simulink model "TCM64QAM_32QAM"  (Simulink 10.2)
settings: Solver=VariableStepDiscrete  StartTime=0.0  StopTime=1000  RelTol=1e-3  EnableMultiTasking=on
model workspace (MAT data in the model file):
  A = 1
  BER_exit = 0.0017398260174
  BER_th = 0.001
  K = 32
  M = 64
  N = 50
  P_TCM = 42
  P_UNCODED = 20.6666666667
  T = 1
  ber_TCM = [0.391236338113 0.382773488419 0.372666198737 0.362839667101 0.34830041111 0.338594204352 0.32505765567 0.309034392861 0.296741201243 0.281058858919 0.266339115612 0.248551087937 0.23457334804 0.215401584278 0.194144189311 0.138453825328 0.0571743708012 0.00563521508072 0.000521407801063 4.01082923895e-05]
  ber_UNCODED = [0.335246475352 0.314468553145 0.294510548945 0.272232776722 0.248595140486 0.22599740026 0.204779522048 0.183241675832 0.16104389561 0.140525947405 0.119748025197 0.10102989701 0.0794720527947 0.0601739826017 0.0424757524248 0.0288171182882 0.0175182481752 0.00995900409959 0.0048195180482 0.0017398260174]
  ber_tcm_bit_coded = [0.48089842575 0.489371302517 0.488168053745 0.487265617166 0.483605735486 0.484508172065 0.484056953775 0.483455329389 0.474029880678 0.474430963602 0.468715531936 0.456582773488 0.44745813697 0.426702095658 0.405444700692 0.320164443999 0.142986062368 0.0183495437682 0.000802165847789 0]
  ber_tcm_bit_uncoded = [0.350234149856 0.340341535072 0.326371459304 0.305454545455 0.28245363766 0.265181458857 0.235078627591 0.191129032258 0.17 0.133428860418 0.104998403066 0.0721370604148 0.0580141843972 0.0456842923795 0.0325443786982 0.0185420832576 0.00556319539942 0.00110539845758 0.000276048986147 5.01353654868e-05]
  coded_bit = 5
  coded_bit_conv = [5 6]
  codegen = [1  0  0  0  0  0; 0  1  0  0  0  0; 0  0  1  0  0  0; 0  0  0  1  0  0; 0  0  0  0  133  171]
  codegen_2 = [133 171]
  constlen = [1 1 1 1 7]
  constlen_2 = 7
  generator_c1 = 133
  generator_c2 = 171
  h = 22
  hh = 0
  hws = Simulink.ModelWorkspace
  i = 21
  k = 5
  label_coded = 'TCM64QAM'
  label_uncoded = '32QAM'
  list : struct (value not decoded)
  m = 6
  mapping_tcm = [-5-5i 3+3i -5+3i 3-5i -1-1i 7+7i -1+7i 7-1i -5-1i 3+7i -5+7i 3-1i -1-5i 7+3i -1+3i 7-5i -7-7i 1+1i -7+1i 1-7i -3-3i 5+5i -3+5i 5-3i -7-3i 1+5i -7+5i 1-3i -3-7i 5+1i -3+1i 5-7i -7-1i 1+7i -7+7i 1-1i -3-5i 5+3i -3+3i 5-5i -7-5i 1+3i -7+3i 1-5i -3-1i 5+7i -3+7i 5-1i -5-3i 3+5i -5+5i 3-3i -1-7i 7+1i -1+1i 7-7i -5-7i 3+1i -5+1i 3-7i -1-3i 7+5i -1+5i 7-3i]
  mdl_name = 'TCM64QAM_32QAM'
  mm = 0
  n = 10000
  num_states = 64
  register_length = 7
  seed = 210846
  snr = 20
  snr_start = 0
  snr_step = 1
  snr_vec = [0 1 2 3 4 5 6 7 8 9 10 11 12 13 14 15 16 17 18 19 20]
  ss = 0.721
  startTime = [2021 6 12 8 25 36.464]
  stepTime = [2021 6 12 8 25 56.984]
  step_dur = 0.721
  tb = 28
  tout = [9001 9002 9003 9004 9005 9006 9007 9008 9009 9010 9011 9012 ... (1000 elements, 1000x1)]
  trellis.numInputSymbols = 32
  trellis.numOutputSymbols = 64
  trellis.numStates = 64
  trellis.nextStates = [0 0 1 1 2 2 3 3 4 4 5 5 ... (2048 elements, 64x32)]
  trellis.outputs = [0 3 2 1 0 3 2 1 3 0 1 2 ... (2048 elements, 64x32)]
  trellis_2.numInputSymbols = 2
  trellis_2.numOutputSymbols = 4
  trellis_2.numStates = 64
  trellis_2.nextStates = [0  32; 0  32; 1  33; 1  33; 2  34; 2  34; 3  35; 3  35; 4  36; 4  36; 5  37; 5  37; 6  38; 6  38; 7  39; 7  39; 8  40; 8  40; 9  41; 9  41; 10  42; 10  42; 11  43; 11  43; 12  44; 12  44; 13  45; 13  45; 14  46; 14  46; 15  47; 15  47; 16  48; 16  48; 17  49; 17  49; 18  50; 18  50; 19  51; 19  51; 20  52; 20  52; 21  53; 21  53; 22  54; 22  54; 23  55; 23  55; 24  56; 24  56; 25  57; 25  57; 26  58; 26  58; 27  59; 27  59; 28  60; 28  60; 29  61; 29  61; 30  62; 30  62; 31  63; 31  63]
  trellis_2.outputs = [0  3; 3  0; 2  1; 1  2; 0  3; 3  0; 2  1; 1  2; 3  0; 0  3; 1  2; 2  1; 3  0; 0  3; 1  2; 2  1; 3  0; 0  3; 1  2; 2  1; 3  0; 0  3; 1  2; 2  1; 0  3; 3  0; 2  1; 1  2; 0  3; 3  0; 2  1; 1  2; 1  2; 2  1; 3  0; 0  3; 1  2; 2  1; 3  0; 0  3; 2  1; 1  2; 0  3; 3  0; 2  1; 1  2; 0  3; 3  0; 2  1; 1  2; 0  3; 3  0; 2  1; 1  2; 0  3; 3  0; 1  2; 2  1; 3  0; 0  3; 1  2; 2  1; 3  0; 0  3]
  uncoded_bit = [1 2 3 4]
undefined symbols (not defined in the file): Mnum
libraries: commsink2 x4, commutil2 x4, dspindex x4, commdigbbndam3 x3, commchan3 x2, commcnvcod2 x2, commdigbbndtcm2 x1, commrandsrc2 x1
settings Model: Creator=Diego  LastModifiedBy=diego
settings DataIOCC: LimitDataPoints=on
settings OptimizationCC: ExpressionDepthLimit=2147483647
settings DebuggingCC: SolverPrmCheckMsg=warning  StateNameClashWarn=warning
settings GRTTargetCC: CombineOutputUpdateFcns=on  GRTInterface=off

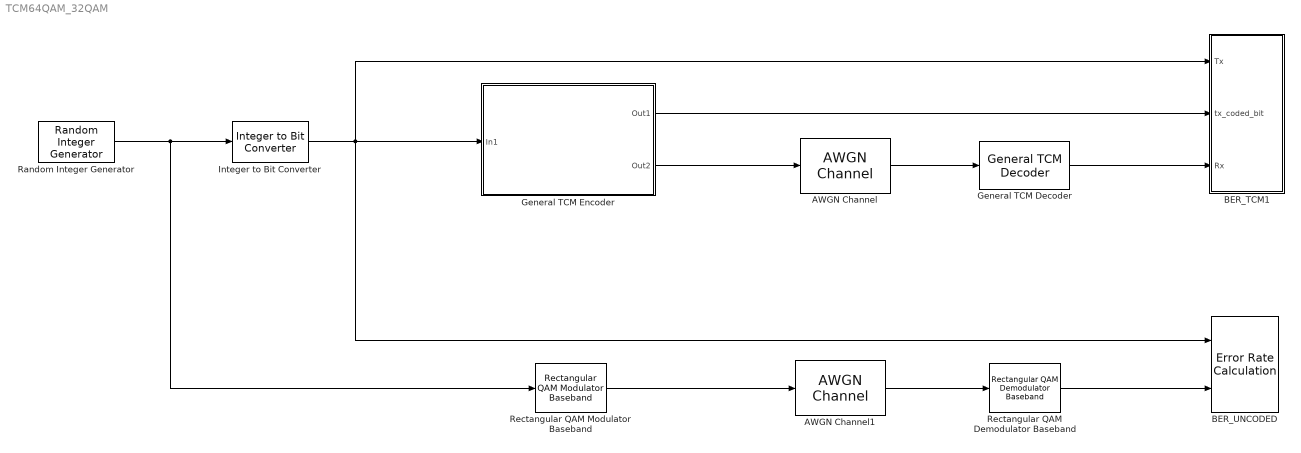
== system TCM64QAM_32QAM ==
  AWGN Channel : commchan3/AWGN Channel  InputProcessing=Columns as channels (frame based)  seed=seed  noiseMode="Signal to noise ratio  (Es/No)"  EbNodB=Eb_No  EsNodB=snr  SNRdB=snr  bitsPerSym=k  Ps=P_TCM  Tsym=T  variance=1
  AWGN Channel1 : commchan3/AWGN Channel  InputProcessing=Columns as channels (frame based)  seed=seed  noiseMode="Signal to noise ratio  (Es/No)"  EbNodB=Eb_No  EsNodB=snr  SNRdB=snr  bitsPerSym=k  Ps=P_UNCODED  Tsym=1  variance=1
  BER_TCM1 : Subsystem
  BER_UNCODED : commsink2/Error Rate Calculation  N=0  st_delay=0  cp_mode=Entire frame  subframe=[]  PMode=Workspace  WsName=ErrorVec_UNCODED  RsMode2=off  stop=off  numErr=100  maxBits=1e6
  General TCM Decoder : commdigbbndtcm2/General TCM Decoder  trellis=trellis  constpts=mapping_tcm  tbdepth=tb  opmode=Continuous  reset=off  outDtype=double
      settings: SourceProductBaseCode=CM
  General TCM Encoder : Subsystem  AncestorBlock=commdigbbndtcm2/General TCM Encoder  mask(General TCM Encoder){trellis=trellis, opMode=Continuous, constpts=mapping_tcm, outDtype=double}
      mask prompts: trellis "Trellis structure:"; opMode "Operation mode:"; constpts "Signal constellation:"; outDtype "Output data type"
      mask help:
      | Convolutionally encode binary data and perform signal mapping using the Signal constellation parameter, which expects complex constellation points in the set-partitioned order.
      |
      | The Trellis structure parameter must be a valid MATLAB trellis structure. To check if a structure is a valid trellis structure, use the istrellis function in MATLAB.
      mask init:
      | [constpts, Mnum, err, inPortLbl, rstPortLbl] = commblkgentcmenc(gcb, 'init', trellis, constpts);
      | if ~isempty(err.msg)
      | 	error(err.mmi,err.msg);
      | end
      mask Help: helpview(commbhelp)
      mask TypeOptions opMode: Continuous | Truncated (reset every frame) | Terminate trellis by appending bits | Reset on nonzero input via port
      mask TypeOptions outDtype: double | single
      mask Callback outDtype: commblkgentcmenc(gcb, 'cbDtype');
      mask Display:
      | disp('General\nTCM');
      | text(inPortLbl.x, inPortLbl.y, inPortLbl.str);
      | text(rstPortLbl.x, rstPortLbl.y, rstPortLbl.str);
  Integer to Bit Converter : commutil2/Integer to Bit Converter  nbits=k  signedInputValues=Unsigned  bitOrder=MSB first  outDtype=Inherit via internal rule
  Random Integer Generator : commrandsrc2/Random Integer Generator  mul=K  seed=seed  Ts=1  frameBased=off  sampPerFrame=frame  orient=off  outDataType=double
      settings: SourceProductBaseCode=CM
  Rectangular QAM Demodulator Baseband : commdigbbndam3/Rectangular QAM Demodulator Baseband  M=K  OutType=Bit  DecType=Hard decision  VarSource=Dialog  Variance=1  Dec=Gray  Mapping=[0:15]  PowType=Min. distance between symbols  MinDist=2  AvgPow=1  PeakPow=1  Ph=0  outDtype1=Inherit via internal rule  outDtype2=Inherit via internal rule  derotateFactorWordLen=16  derotateFactorDataTypeStr=Inherit: Same word length as input  derotateFactorLastDataTypeStr=Inherit: Same word length as input  denormFactorWordLen=16  denormFactorDataTypeStr=Inherit: Same word length as input  denormFactorLastDataTypeStr=Inherit: Same word length as input  prodOutWordLen=32  prodOutOverflowMode=Wrap  prodOutRoundingMode=Floor  prodOutOvFlMode=off  prodOutOvFlModeLastStrValue=off  sumWordLen=32
  Rectangular QAM Modulator Baseband : commdigbbndam3/Rectangular QAM Modulator Baseband  M=K  InType=Integer  Enc=Gray  Mapping=[0:15]  PowType=Min. distance between symbols  MinDist=2  AvgPow=1  PeakPow=1  Ph=0  outDtype=double  outWordLen=16  outUDDataType=sfix(16)  outFracLenMode=Best precision  outFracLen=15  outDataTypeStr=double  outLastDataTypeStr=double
  wires:
  Random Integer Generator/1 -> Integer to Bit Converter/1, Rectangular QAM Modulator Baseband/1
  Integer to Bit Converter/1 -> BER_UNCODED/1, General TCM Encoder/1(In1), BER_TCM1/1(Tx)
  General TCM Encoder/2(Out2) -> AWGN Channel/1
  AWGN Channel/1 -> General TCM Decoder/1
  Rectangular QAM Modulator Baseband/1 -> AWGN Channel1/1
  AWGN Channel1/1 -> Rectangular QAM Demodulator Baseband/1
  Rectangular QAM Demodulator Baseband/1 -> BER_UNCODED/2
  General TCM Decoder/1 -> BER_TCM1/3(Rx)
  General TCM Encoder/1(Out1) -> BER_TCM1/2(tx_coded_bit)

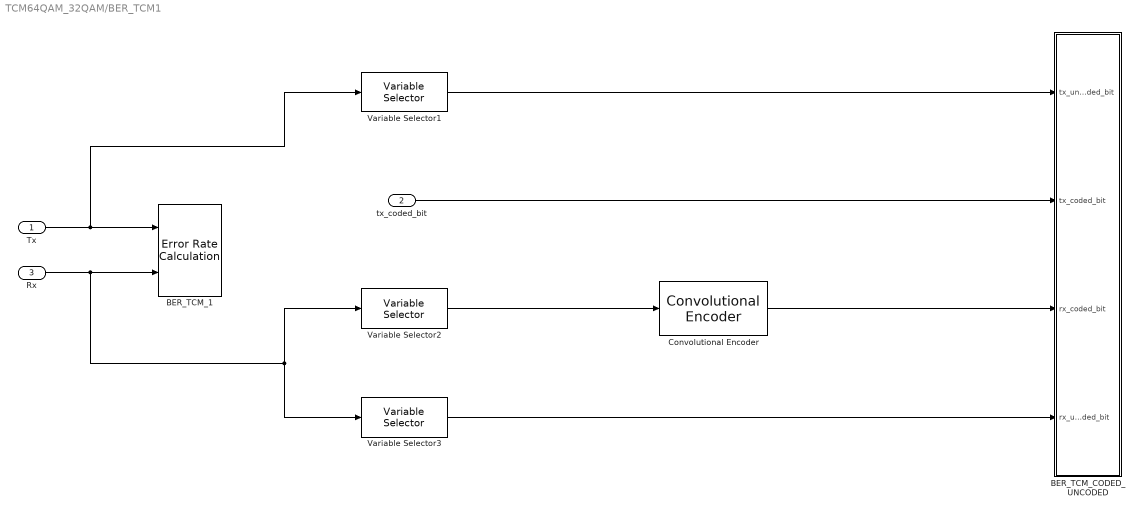
== system TCM64QAM_32QAM/BER_TCM1 ==
  Tx : Inport
  tx_coded_bit : Inport  Port=2
  Rx : Inport  Port=3
  BER_TCM_1 : commsink2/Error Rate Calculation  N=tb*k  st_delay=0  cp_mode=Entire frame  subframe=[]  PMode=Workspace  WsName=ErrorVec_TCM_1  RsMode2=off  stop=off  numErr=100  maxBits=1e6
  BER_TCM_CODED_UNCODED : Subsystem
  Convolutional Encoder : commcnvcod2/Convolutional Encoder  trellis=trellis_2  opMode=Continuous  DelayedResetAction=off  hasIniStPort=off  hasFinStPort=off  usePuncVector=off  punctureVector=[1; 1; 0; 1; 0; 1]  reset=Unused parameter value
      settings: SourceProductBaseCode=CM
  Variable Selector1 : dspindex/Variable Selector  NumInputs=1  rowsOrCols=Rows  IdxMode=Fixed  Elements=uncoded_bit  ZerOneIdxMode=One-based  errmode=Clip Index  FillMode=on  FillValues=0
  Variable Selector2 : dspindex/Variable Selector  NumInputs=1  rowsOrCols=Rows  IdxMode=Fixed  Elements=coded_bit  ZerOneIdxMode=One-based  errmode=Clip Index  FillMode=on  FillValues=0
  Variable Selector3 : dspindex/Variable Selector  NumInputs=1  rowsOrCols=Rows  IdxMode=Fixed  Elements=uncoded_bit  ZerOneIdxMode=One-based  errmode=Clip Index  FillMode=on  FillValues=0
  wires:
  Tx/1 -> BER_TCM_1/1, Variable Selector1/1
  Rx/1 -> BER_TCM_1/2, Variable Selector2/1, Variable Selector3/1
  Variable Selector1/1 -> BER_TCM_CODED_UNCODED/1(tx_uncoded_bit)
  Variable Selector2/1 -> Convolutional Encoder/1
  Variable Selector3/1 -> BER_TCM_CODED_UNCODED/4(rx_uncoded_bit)
  tx_coded_bit/1 -> BER_TCM_CODED_UNCODED/2(tx_coded_bit)
  Convolutional Encoder/1 -> BER_TCM_CODED_UNCODED/3(rx_coded_bit)

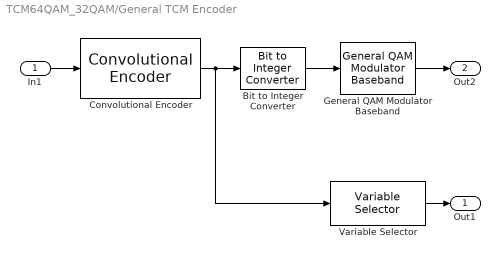
== system TCM64QAM_32QAM/General TCM Encoder ==
  In1 : Inport
  Bit to Integer Converter : commutil2/Bit to Integer Converter  nbits=log2(Mnum)  bitOrder=MSB first  signedOutputValues=Unsigned  outDtype=uint32  outDtypeSigned=Inherit via internal rule
  Convolutional Encoder : commcnvcod2/Convolutional Encoder  trellis=trellis  opMode=Continuous  DelayedResetAction=off  hasIniStPort=off  hasFinStPort=off  usePuncVector=off  punctureVector=[1; 1; 0; 1; 0; 1]  reset=Unused parameter value
      settings: SourceProductBaseCode=CM
  General QAM Modulator Baseband : commdigbbndam3/General QAM Modulator Baseband  SigCon=constpts  outDtype=double  outWordLen=16  outUDDataType=sfix(16)  outFracLenMode=Best precision  outFracLen=15  outDataTypeStr=double  outLastDataTypeStr=double
      settings: SourceProductBaseCode=CM
  Variable Selector : dspindex/Variable Selector  NumInputs=1  rowsOrCols=Rows  IdxMode=Fixed  Elements=coded_bit_conv  ZerOneIdxMode=One-based  errmode=Clip Index  FillMode=on  FillValues=0
  Out1 : Outport
  Out2 : Outport  Port=2
  wires:
  Bit to Integer Converter/1 -> General QAM Modulator Baseband/1
  In1/1 -> Convolutional Encoder/1
  Convolutional Encoder/1 -> Bit to Integer Converter/1, Variable Selector/1
  General QAM Modulator Baseband/1 -> Out2/1
  Variable Selector/1 -> Out1/1

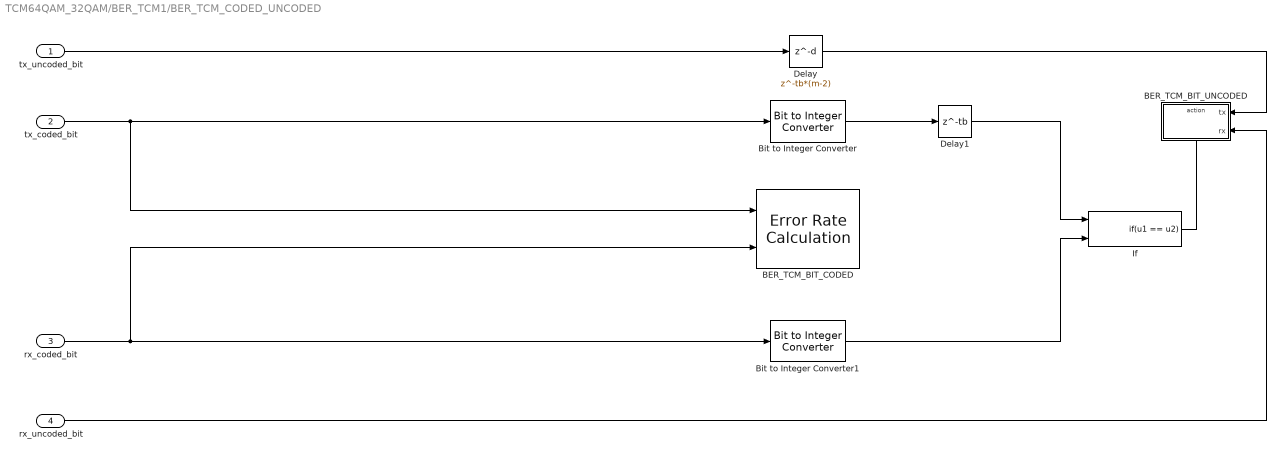
== system TCM64QAM_32QAM/BER_TCM1/BER_TCM_CODED_UNCODED ==
  tx_uncoded_bit : Inport
  tx_coded_bit : Inport  Port=2
  rx_coded_bit : Inport  Port=3
  rx_uncoded_bit : Inport  Port=4
  BER_TCM_BIT_CODED : commsink2/Error Rate Calculation  N=tb*2  st_delay=0  cp_mode=Entire frame  subframe=[]  PMode=Workspace  WsName=ErrorVec_TCM_COD_1  RsMode2=off  stop=off  numErr=100  maxBits=1e6
  BER_TCM_BIT_UNCODED : Subsystem  TreatAsAtomicUnit=on
  Bit to Integer Converter : commutil2/Bit to Integer Converter  nbits=2  bitOrder=MSB first  signedOutputValues=Unsigned  outDtype=Inherit via internal rule  outDtypeSigned=Inherit via internal rule
  Bit to Integer Converter1 : commutil2/Bit to Integer Converter  nbits=2  bitOrder=MSB first  signedOutputValues=Unsigned  outDtype=Inherit via internal rule  outDtypeSigned=Inherit via internal rule
  Delay : Delay  DelayLength=tb*(m-2)  InputProcessing=Columns as channels (frame based)
  Delay1 : Delay  DelayLength=tb  InputProcessing=Columns as channels (frame based)
  If : If  NumInputs=2  IfExpression=u1 == u2  ShowElse=off
  wires:
  tx_uncoded_bit/1 -> Delay/1
  tx_coded_bit/1 -> BER_TCM_BIT_CODED/1, Bit to Integer Converter/1
  rx_coded_bit/1 -> BER_TCM_BIT_CODED/2, Bit to Integer Converter1/1
  Delay/1 -> BER_TCM_BIT_UNCODED/1(tx)
  rx_uncoded_bit/1 -> BER_TCM_BIT_UNCODED/2(rx)
  If/1 -> BER_TCM_BIT_UNCODED/Action
  Bit to Integer Converter/1 -> Delay1/1
  Bit to Integer Converter1/1 -> If/2
  Delay1/1 -> If/1

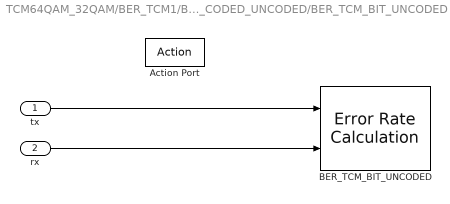
== system TCM64QAM_32QAM/BER_TCM1/BER_TCM_CODED_UNCODED/BER_TCM_BIT_UNCODED ==
  tx : Inport
  rx : Inport  Port=2
  Action Port : ActionPort  ActionPortLabel=if(u1 == u2)
  BER_TCM_BIT_UNCODED : commsink2/Error Rate Calculation  N=0  st_delay=tb*(m-2)  cp_mode=Entire frame  subframe=[]  PMode=Workspace  WsName=ErrorVec_TCM_bit_uncoded  RsMode2=off  stop=off  numErr=100  maxBits=1e6
  wires:
  tx/1 -> BER_TCM_BIT_UNCODED/1
  rx/1 -> BER_TCM_BIT_UNCODED/2
